simulink model "LS_Variables"  (R2015a)
settings: Solver=ode45  StartTime=0.0  StopTime=10.0  RelTol=1e-3
undefined symbols (not defined in the file or in its folder): dist, lat, lon, theta
settings Model: Creator=John  LastModifiedBy=John

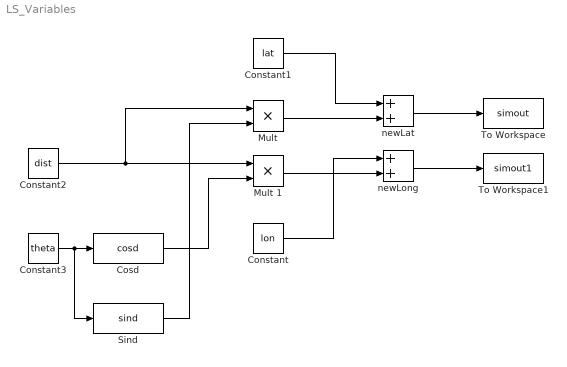
== system LS_Variables ==
  Constant : Constant  Value=lon
  Constant1 : Constant  Value=lat
  Constant2 : Constant  Value=dist
  Constant3 : Constant  Value=theta
  "Cosd " : MATLABFcn  MATLABFcn=cosd
  "Mult " : Product  Inputs=**
  Mult 1 : Product  Inputs=**
  "Sind " : MATLABFcn  MATLABFcn=sind
  To Workspace : ToWorkspace  VariableName=simout  SaveFormat=Timeseries  SampleTime=-1
  To Workspace1 : ToWorkspace  VariableName=simout1  SaveFormat=Timeseries  SampleTime=-1
  newLat : Sum
  newLong : Sum
  wires:
  Constant3/1 -> "Sind "/1, "Cosd "/1
  "Cosd "/1 -> Mult 1/2
  "Sind "/1 -> "Mult "/2
  Constant2/1 -> "Mult "/1, Mult 1/1
  Mult 1/1 -> newLong/2
  Constant/1 -> newLong/1
  "Mult "/1 -> newLat/2
  Constant1/1 -> newLat/1
  newLat/1 -> To Workspace/1
  newLong/1 -> To Workspace1/1
